simulink model "task_2_sim"  (R2023a)
settings: Solver=VariableStepAuto  StartTime=0.0  StopTime=25  MaxStep=1e-4  RelTol=1e-4
undefined symbols (not defined in the file): A, B, Bw, C, C_Z, D_Z, Dw, K, L, x0
settings Model: Creator=user  LastModifiedBy=user

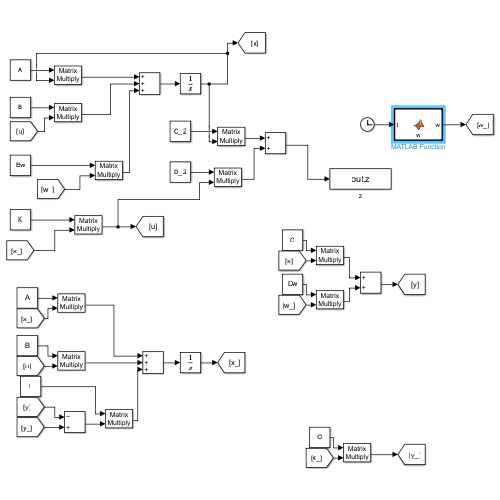
[thumbnail: Simulink's stored preview of the top-level diagram]
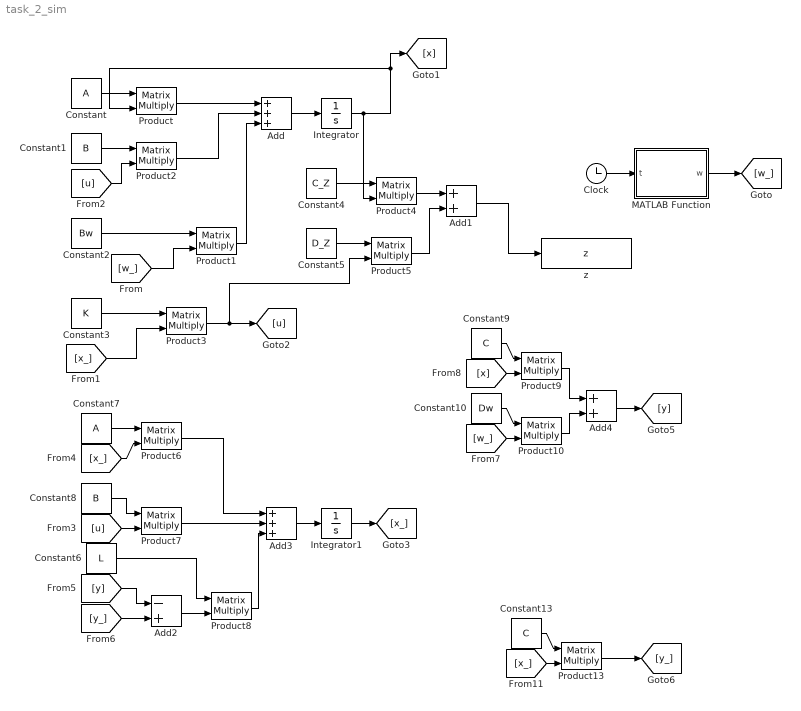
== system task_2_sim ==
  Add : Sum  Inputs=+++
  Add1 : Sum
  Add2 : Sum  Inputs=-+
  Add3 : Sum  Inputs=+++
  Add4 : Sum
  Clock : Clock
  Constant : Constant  Value=A  VectorParams1D=off
  Constant1 : Constant  Value=B  VectorParams1D=off
  Constant10 : Constant  Value=Dw  VectorParams1D=off
  Constant13 : Constant  Value=C  VectorParams1D=off
  Constant2 : Constant  Value=Bw  VectorParams1D=off
  Constant3 : Constant  Value=K  VectorParams1D=off
  Constant4 : Constant  Value=C_Z  VectorParams1D=off
  Constant5 : Constant  Value=D_Z  VectorParams1D=off
  Constant6 : Constant  Value=L  VectorParams1D=off
  Constant7 : Constant  Value=A  VectorParams1D=off
  Constant8 : Constant  Value=B  VectorParams1D=off
  Constant9 : Constant  Value=C  VectorParams1D=off
  Integrator : Integrator  InitialCondition=x0
  Integrator1 : Integrator  InitialCondition=x0
  MATLAB Function : MATLAB Function  TreatAsAtomicUnit=on
  Product{,1..10,13} (12 alike) : Product  Multiplication=Matrix(*)
  z : ToWorkspace  VariableName=z  SaveFormat=Timeseries  SampleTime=-1
  wires:
  Clock/1 -> MATLAB Function/1(t)
  MATLAB Function/1(w) -> [w_]
  Integrator/1 -> Product4/2, Product/2, [x]
  Constant/1 -> Product/1
  Add/1 -> Integrator/1
  Product/1 -> Add/1
  Constant3/1 -> Product3/1
  [x_] -> Product3/2
  Product3/1 -> Product5/2, [u]
  Constant1/1 -> Product2/1
  [u] -> Product2/2
  Product2/1 -> Add/2
  Constant2/1 -> Product1/1
  [w_] -> Product1/2
  Product1/1 -> Add/3
  Constant4/1 -> Product4/1
  Constant5/1 -> Product5/1
  Product5/1 -> Add1/2
  Product4/1 -> Add1/1
  Add1/1 -> z/1
  Constant7/1 -> Product6/1
  [x_] -> Product6/2
  [u] -> Product7/2
  Constant8/1 -> Product7/1
  [y] -> Add2/1
  [y_] -> Add2/2
  Add2/1 -> Product8/2
  Constant6/1 -> Product8/1
  Product6/1 -> Add3/1
  Product7/1 -> Add3/2
  Product8/1 -> Add3/3
  Add3/1 -> Integrator1/1
  Integrator1/1 -> [x_]
  [w_] -> Product10/2
  Constant10/1 -> Product10/1
  Constant9/1 -> Product9/1
  [x] -> Product9/2
  Product9/1 -> Add4/1
  Product10/1 -> Add4/2
  Add4/1 -> [y]
  Constant13/1 -> Product13/1
  [x_] -> Product13/2
  Product13/1 -> [y_]

== matlab function task_2_sim/MATLAB Function ==
  data: t input; w output
function w = w(t)
    w = [sin(0.7*t);
         0];
    
end
